simulink model "simulation_input_constraint"  (R2023b)
settings: Solver=VariableStepAuto  StartTime=0  StopTime=t_end  RelTol=1e-3
InitFcn:
  | param = plant_param();
values from neighbouring files (symbols this model uses):
  t_end = (N-1)*Ts    [plot_bode.m]
libraries: fl_lib x8, nesl_utility x7, simulink x1
(part 1 of 3)
settings Model: Creator=block  LastModifiedBy=block
settings DataIOCC: SaveFormat=StructureWithTime
settings OptimizationCC: BlockReduction=off  BufferReuse=off
settings DebuggingCC: AlgebraicLoopMsg=none

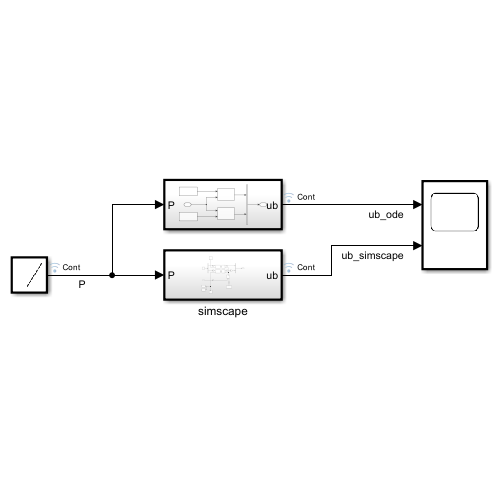
[thumbnail: Simulink's stored preview of the top-level diagram]
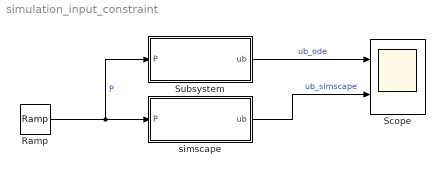
== system simulation_input_constraint ==
  Ramp : simulink/Sources/Ramp  slope=2*param.Ps/t_end  start=0  InitialOutput=10
  Scope : Scope  NumInputPorts=2
  Subsystem : Subsystem
  simscape : Subsystem
  wires:
  Subsystem/1(ub) -> Scope/1  "ub_ode"
  simscape/1(ub) -> Scope/2  "ub_simscape"
  Ramp/1 -> Subsystem/1(P), simscape/1(P)  "P"

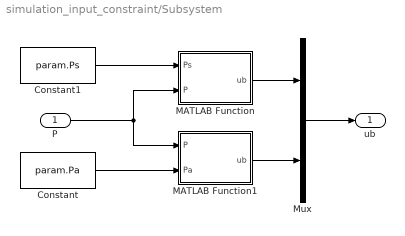
== system simulation_input_constraint/Subsystem ==
  P : Inport
  Constant : Constant  Value=param.Pa
  Constant1 : Constant  Value=param.Ps
  MATLAB Function : MATLAB Function  TreatAsAtomicUnit=on
  MATLAB Function1 : MATLAB Function  TreatAsAtomicUnit=on
  Mux : Mux  Inputs=2
  ub : Outport
  wires:
  P/1 -> MATLAB Function1/1(P), MATLAB Function/2(P)
  Constant1/1 -> MATLAB Function/1(Ps)
  Constant/1 -> MATLAB Function1/2(Pa)
  MATLAB Function/1(ub) -> Mux/1
  MATLAB Function1/1(ub) -> Mux/2
  Mux/1 -> ub/1
